simulink model "Subsystem"  (R2020a)
settings: Solver=VariableStepAuto  StartTime=0.0  StopTime=10.0  RelTol=1e-3
values from neighbouring files (symbols this model uses):
  I = 5.0    [AbsData.sldd]
  Kf = 1.0    [AbsData.sldd]
  PBmax = 1500.0    [AbsData.sldd]
  Rr = 1.25    [AbsData.sldd]
  TB = 0.01    [AbsData.sldd]
  v0 = 88.0    [AbsData.sldd]
settings Model: DataDictionary=AbsData.sldd  Creator=kasutav  LastModifiedBy=kasutav
settings DataIOCC: SaveOutput=off  SaveTime=off

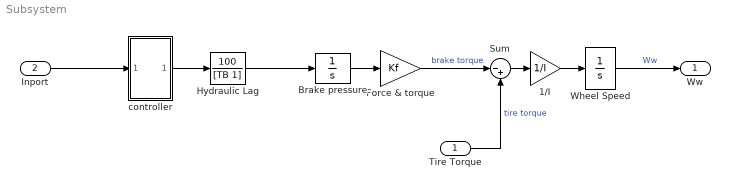
== system Subsystem ==
  Tire Torque : Inport  OutDataTypeStr=double  PortDimensions=1  SampleTime=0
  Inport : Inport  Port=2  OutDataTypeStr=double  PortDimensions=1  SampleTime=0
  1/I : Gain  Gain=1/I  SaturateOnIntegerOverflow=on  OutDataTypeStr=Inherit: Same as input  ParamDataTypeStr=Inherit: Same as input
  Brake pressure : Integrator  LimitOutput=on  UpperSaturationLimit=PBmax  LowerSaturationLimit=0
  Force & torque : Gain  Gain=Kf  SaturateOnIntegerOverflow=on  OutDataTypeStr=Inherit: Same as input  ParamDataTypeStr=Inherit: Same as input
  "Hydraulic Lag " : TransferFcn  Numerator=[100]  Denominator=[TB 1]
  Sum : Sum  Inputs=|-+  InputSameDT=on  SaturateOnIntegerOverflow=on  OutDataTypeStr=Inherit: Same as first input
  Wheel Speed : Integrator  InitialCondition=v0/Rr  LimitOutput=on  UpperSaturationLimit=1000  LowerSaturationLimit=0
  "controller " : Subsystem
  Ww : Outport  OutDataTypeStr=double  PortDimensions=1  SampleTime=0
  wires:
  Inport/1 -> "controller "/1(Inport)
  1/I/1 -> Wheel Speed/1
  "Hydraulic Lag "/1 -> Brake pressure/1
  Wheel Speed/1 -> Ww/1  "Ww"
  Force & torque/1 -> Sum/1  "brake torque"
  "controller "/1(Out1) -> "Hydraulic Lag "/1
  Tire Torque/1 -> Sum/2  "tire torque"
  Brake pressure/1 -> Force & torque/1
  Sum/1 -> 1/I/1

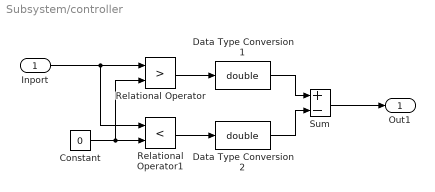
== system Subsystem/controller  ==
  Inport : Inport
  Constant : Constant  Value=0
  Data Type Conversion1 : DataTypeConversion  OutDataTypeStr=double  SaturateOnIntegerOverflow=on  RndMeth=Zero
  Data Type Conversion2 : DataTypeConversion  OutDataTypeStr=double  SaturateOnIntegerOverflow=on  RndMeth=Zero
  Relational Operator : RelationalOperator  Operator=>  OutDataTypeStr=boolean  RndMeth=Nearest  InputSameDT=on
  Relational Operator1 : RelationalOperator  Operator=<  OutDataTypeStr=boolean  RndMeth=Nearest  InputSameDT=on
  Sum : Sum  Inputs=+-  InputSameDT=on  SaturateOnIntegerOverflow=on  OutDataTypeStr=Inherit: Same as first input
  Out1 : Outport
  wires:
  Constant/1 -> Relational Operator1/2, Relational Operator/2
  Data Type Conversion1/1 -> Sum/1
  Data Type Conversion2/1 -> Sum/2
  Relational Operator/1 -> Data Type Conversion1/1
  Inport/1 -> Relational Operator/1, Relational Operator1/1
  Relational Operator1/1 -> Data Type Conversion2/1
  Sum/1 -> Out1/1
